simulink model "Discrete_PID"  (R2016a)
settings: Solver=ode45  StartTime=0.0  StopTime=10.0  RelTol=1e-3
settings Model: Creator=admin  LastModifiedBy=admin

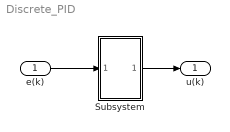
== system Discrete_PID ==
  e(k) : Inport
  Subsystem : Subsystem  mask{Kp=0, Ki=0, Kd=0, T=0.001, U_m=10}
      mask prompts: Kp "Proportional Kp"; Ki "Integrator Ki"; Kd "Derivative Kd"; T "Sampling period T"; U_m "limit"
      mask Display: disp('Discrete PID')
  "u(k) " : Outport
  wires:
  e(k)/1 -> Subsystem/1(e(k))
  Subsystem/1("u(k) ") -> "u(k) "/1

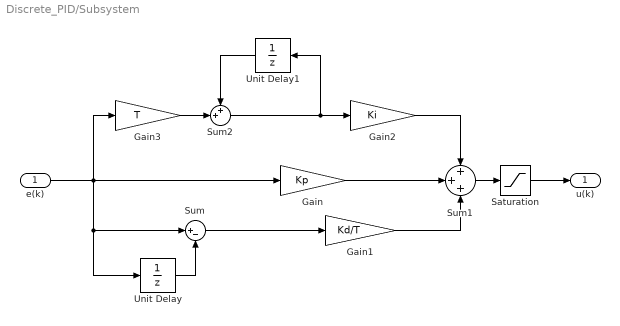
== system Discrete_PID/Subsystem ==
  e(k) : Inport
  Gain : Gain  Gain=Kp
  Gain1 : Gain  Gain=Kd/T
  Gain2 : Gain  Gain=Ki
  Gain3 : Gain  Gain=T
  Saturation : Saturate  UpperLimit=U_m  LowerLimit=-U_m
  Sum : Sum  Inputs=|+-
  Sum1 : Sum  Inputs=+++
  Sum2 : Sum  Inputs=++|
  Unit Delay : UnitDelay  SampleTime=-1
  Unit Delay1 : UnitDelay  SampleTime=-1
  "u(k) " : Outport
  wires:
  Sum/1 -> Gain1/1
  Unit Delay1/1 -> Sum2/1
  Sum2/1 -> Unit Delay1/1, Gain2/1
  Gain3/1 -> Sum2/2
  Gain1/1 -> Sum1/3
  Saturation/1 -> "u(k) "/1
  e(k)/1 -> Gain3/1, Gain/1, Sum/1, Unit Delay/1
  Sum1/1 -> Saturation/1
  Unit Delay/1 -> Sum/2
  Gain/1 -> Sum1/2
  Gain2/1 -> Sum1/1
